simulink model "double_inverted_pendulum3"  (R2021b)
settings: Solver=VariableStepAuto  StartTime=0.0  StopTime=20  RelTol=1e-3
libraries: mpclib x1
settings Model: Creator=Dev Vaibhav  LastModifiedBy=Dev Vaibhav

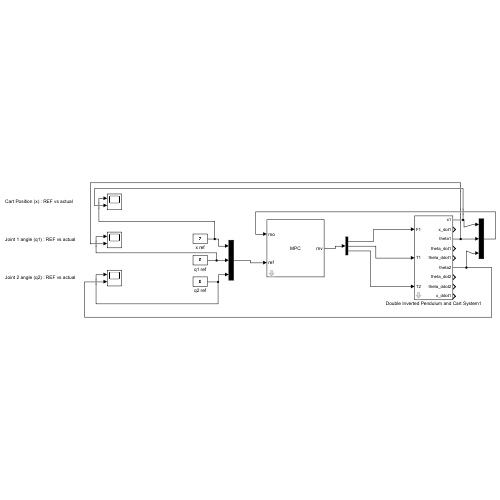
[thumbnail: Simulink's stored preview of the top-level diagram]
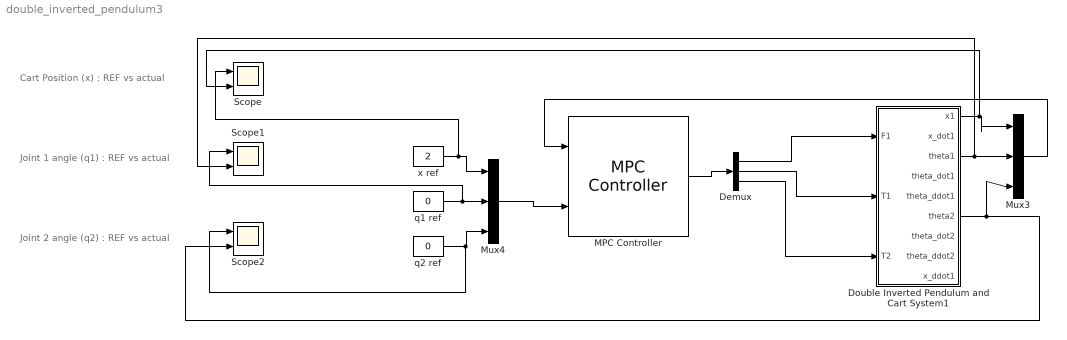
== system double_inverted_pendulum3 ==
  note: Cart Position (x) : REF vs actual
  note: Joint 1 angle (q1) : REF vs actual
  note: Joint 2 angle (q2) : REF vs actual
  Demux : Demux  Outputs=3
  Double Inverted Pendulum and Cart System1 : Subsystem  mask{mCartPara=1, mPendPara=1, gPara=9.81, LPara=0.5, KdPara=10}
      mask prompts: mCartPara "Mass of Cart"; mPendPara "Mass of Pendulum"; gPara "Gravity"; LPara "Length of Pendulum"; KdPara "Friction coefficient of Cart"
      mask help: Pendulum and Cart System
      mask init:
      | mCart = str2double(get_param(gcb,'mCartPara'));
      | mPend = str2double(get_param(gcb,'mPendPara'));
      | g = str2double(get_param(gcb,'gPara'));
      | L = str2double(get_param(gcb,'LPara'));
      | Kd = str2double(get_param(gcb,'KdPara'));
  MPC Controller : mpclib/MPC Controller  SCDEnableBlockLinearizationSpecification=on  mpcobj=mpc1  is_multiple=0  enable_value=0  return_u0=off  updateMPCinCallerWorkspace=on  md_inport=off  mv_inport=off  uref_inport=off  return_cost=off  return_mvseq=off  return_qpstatus=off  return_xseq=off  return_state=off  return_ovseq=off  state_inport=off  umin_inport=off  umax_inport=off  ymin_inport=off  ymax_inport=off  cc_inport=off  ywt_inport=off  uwt_inport=off  duwt_inport=off  rhoeps_inport=off  pm_inport=off  MaximumP=10  HorizonChoice=FixedHorizon  n_ts=0.05  n_p=13  n_mv=3  n_md=0  n_ud=0  n_mo=3  n_uo=0  BlockDataType=double  SampleTimeInherited=off  switch_inport=off
  Mux3 : Mux  Inputs=3
  Mux4 : Mux  Inputs=3
  Scope : Scope  NumInputPorts=2
  Scope1 : Scope  NumInputPorts=2
  Scope2 : Scope  NumInputPorts=2
  q1 ref : Constant  Value=0
  q2 ref : Constant  Value=0
  x ref : Constant  Value=2
  wires:
  q1 ref/1 -> Scope1/1, Mux4/2
  Demux/3 -> Double Inverted Pendulum and Cart System1/3(T2)
  MPC Controller/1 -> Demux/1
  Mux3/1 -> MPC Controller/1
  Demux/2 -> Double Inverted Pendulum and Cart System1/2(T1)
  Demux/1 -> Double Inverted Pendulum and Cart System1/1(F1)
  Double Inverted Pendulum and Cart System1/1(x1) -> Scope/2, Mux3/1
  Double Inverted Pendulum and Cart System1/3(theta1) -> Scope1/2, Mux3/2
  q2 ref/1 -> Scope2/1, Mux4/3
  Mux4/1 -> MPC Controller/2
  x ref/1 -> Scope/1, Mux4/1
  Double Inverted Pendulum and Cart System1/6(theta2) -> Scope2/2, Mux3/3

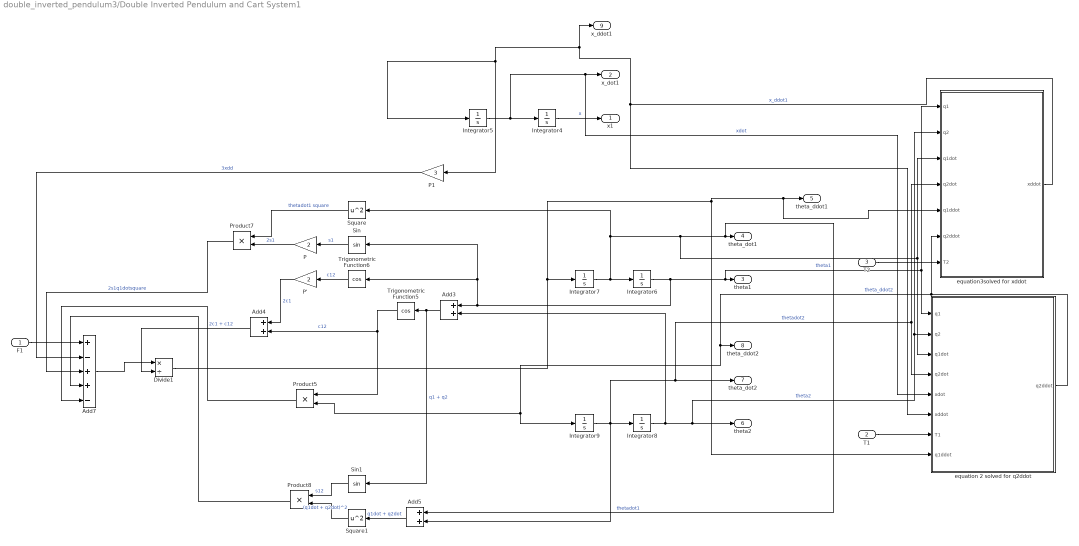
== system double_inverted_pendulum3/Double Inverted Pendulum and Cart System1 ==
  F1 : Inport
  T1 : Inport  Port=2
  T2 : Inport  Port=3
  Add3 : Sum
  Add4 : Sum
  Add5 : Sum
  Add7 : Sum  Inputs=+-++-
  Divide1 : Product  Inputs=*/
  Integrator4 : Integrator  ContinuousStateAttributes='x'
  Integrator5 : Integrator  ContinuousStateAttributes='xdot'
  Integrator6 : Integrator  ContinuousStateAttributes='theta'
  Integrator7 : Integrator  ContinuousStateAttributes='thetadot'
  Integrator8 : Integrator  ContinuousStateAttributes='theta'
  Integrator9 : Integrator  ContinuousStateAttributes='thetadot'
  P : Gain  Gain=2
  P' : Gain  Gain=2
  P1 : Gain  Gain=3
  Product5 : Product
  Product7 : Product
  Product8 : Product
  Sin : Trigonometry
  Sin1 : Trigonometry
  Square : Math  Operator=square  SaturateOnIntegerOverflow=on
  Square1 : Math  Operator=square  SaturateOnIntegerOverflow=on
  Trigonometric Function5 : Trigonometry  Operator=cos
  Trigonometric Function6 : Trigonometry  Operator=cos
  equation 2 solved for q2ddot : Subsystem
  equation3solved for xddot : Subsystem
  x1 : Outport  VectorParamsAs1DForOutWhenUnconnected=off
  x_dot1 : Outport  Port=2  VectorParamsAs1DForOutWhenUnconnected=off
  theta1 : Outport  Port=3  VectorParamsAs1DForOutWhenUnconnected=off
  theta_dot1 : Outport  Port=4  VectorParamsAs1DForOutWhenUnconnected=off
  theta_ddot1 : Outport  Port=5  VectorParamsAs1DForOutWhenUnconnected=off
  theta2 : Outport  Port=6  VectorParamsAs1DForOutWhenUnconnected=off
  theta_dot2 : Outport  Port=7  VectorParamsAs1DForOutWhenUnconnected=off
  theta_ddot2 : Outport  Port=8  VectorParamsAs1DForOutWhenUnconnected=off
  x_ddot1 : Outport  Port=9  VectorParamsAs1DForOutWhenUnconnected=off
  wires:
  Integrator7/1 -> Integrator6/1, Square/1, equation3solved for xddot/3(q1dot), equation 2 solved for q2ddot/3(q1dot), Add5/1, theta_dot1/1  "thetadot1"
  equation3solved for xddot/1(xddot) -> P1/1, Integrator5/1, x_ddot1/1, equation 2 solved for q2ddot/6(xddot)  "x_ddot1"
  Integrator5/1 -> equation 2 solved for q2ddot/5(xdot), x_dot1/1, Integrator4/1  "xdot"
  Integrator6/1 -> Sin/1, Trigonometric Function6/1, Add3/1, equation 2 solved for q2ddot/1(q1), equation3solved for xddot/1(q1), theta1/1  "theta1"
  Integrator4/1 -> x1/1  "x"
  Integrator9/1 -> Add5/2, Integrator8/1, equation3solved for xddot/4(q2dot), equation 2 solved for q2ddot/4(q2dot), theta_dot2/1  "thetadot2"
  Integrator8/1 -> Add3/2, equation3solved for xddot/2(q2), equation 2 solved for q2ddot/2(q2), theta2/1  "theta2"
  equation 2 solved for q2ddot/1(q2ddot) -> Integrator9/1, Product5/2, theta_ddot2/1, equation3solved for xddot/6(q2ddot)  "theta_ddot2"
  Add3/1 -> Sin1/1, Trigonometric Function5/1  "q1 + q2"
  Trigonometric Function5/1 -> Add4/2, Product5/1  "c12"
  Trigonometric Function6/1 -> P'/1  "c12"
  P'/1 -> Add4/1  "2c1"
  Sin/1 -> P/1  "s1"
  P/1 -> Product7/2  "2s1"
  Square/1 -> Product7/1  "thetadot1 square"
  Add5/1 -> Square1/1  "q1dot + q2dot"
  Square1/1 -> Product8/2  "(q1dot + q2dot)^2"
  Sin1/1 -> Product8/1  "s12"
  Product8/1 -> Add7/4
  Product7/1 -> Add7/3  "2s1q1dotsquare"
  F1/1 -> Add7/1
  P1/1 -> Add7/2  "3xdd"
  Product5/1 -> Add7/5
  Add7/1 -> Divide1/1
  Add4/1 -> Divide1/2  "2c1 + c12"
  T1/1 -> equation 2 solved for q2ddot/7(T1)
  T2/1 -> equation3solved for xddot/7(T2)
  Divide1/1 -> equation 2 solved for q2ddot/8(q1ddot), equation3solved for xddot/5(q1ddot), theta_ddot1/1, Integrator7/1

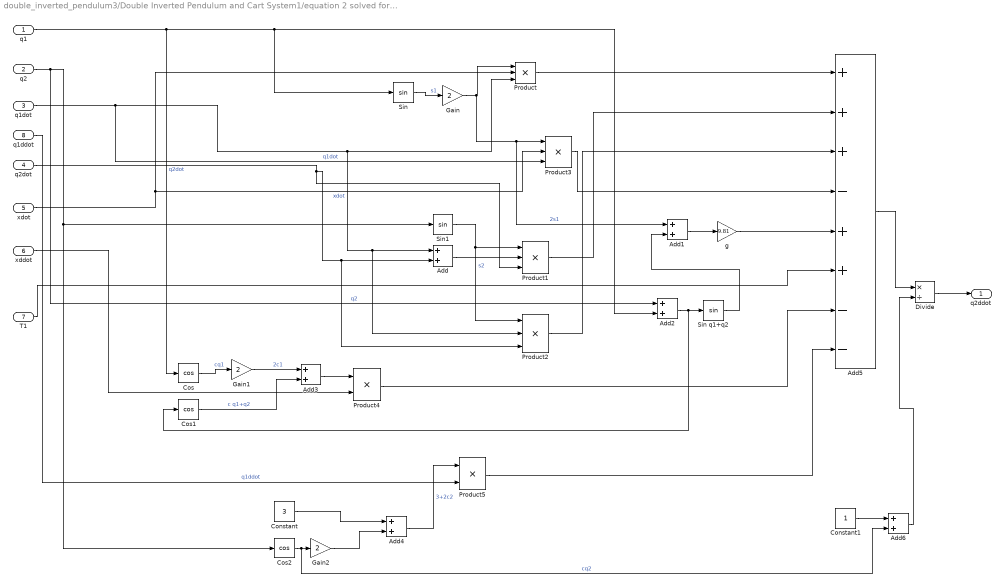
== system double_inverted_pendulum3/Double Inverted Pendulum and Cart System1/equation 2 solved for q2ddot ==
  q1 : Inport
  q2 : Inport  Port=2
  q1dot : Inport  Port=3
  q2dot : Inport  Port=4
  xdot : Inport  Port=5
  xddot : Inport  Port=6
  T1 : Inport  Port=7
  q1ddot : Inport  Port=8
  Add{,1..4,6} (6 alike) : Sum
  Add5 : Sum  Inputs=+++-++--
  Constant : Constant  Value=3
  Constant1 : Constant
  Cos : Trigonometry  Operator=cos
  Cos1 : Trigonometry  Operator=cos
  Cos2 : Trigonometry  Operator=cos
  Divide : Product  Inputs=*/
  Gain : Gain  Gain=2
  Gain1 : Gain  Gain=2
  Gain2 : Gain  Gain=2
  Product{,1..3} (4 alike) : Product  Inputs=3
  Product4 : Product
  Product5 : Product
  Sin : Trigonometry
  Sin q1+q2 : Trigonometry
  Sin1 : Trigonometry
  g : Gain  Gain=9.81
  q2ddot : Outport
  wires:
  q1/1 -> Cos/1, Add2/2, Sin/1
  Sin/1 -> Gain/1  "s1"
  Gain/1 -> Add1/1, Product3/1, Product/1  "2s1"
  xdot/1 -> Product3/2, Product/2  "xdot"
  q2/1 -> Add2/1, Cos2/1, Sin1/1  "q2"
  q2dot/1 -> Product1/3, Product2/3, Add/2  "q2dot"
  Sin1/1 -> Product2/1, Product1/1  "s2"
  Add/1 -> Product1/2
  q1dot/1 -> Product3/3, Product2/2, Add/1, Product/3  "q1dot"
  Add2/1 -> Cos1/1, Sin q1+q2/1
  Sin q1+q2/1 -> Add1/2
  Add1/1 -> g/1
  Cos/1 -> Gain1/1  "cq1"
  Gain1/1 -> Add3/1  "2c1"
  Cos1/1 -> Add3/2  "c q1+q2"
  Add3/1 -> Product4/1
  xddot/1 -> Product4/2
  Cos2/1 -> Add6/2, Gain2/1  "cq2"
  Constant/1 -> Add4/1
  Gain2/1 -> Add4/2
  Add4/1 -> Product5/1  "3+2c2"
  q1ddot/1 -> Product5/2  "q1ddot"
  Product/1 -> Add5/1
  Product1/1 -> Add5/2
  Product2/1 -> Add5/3
  Product3/1 -> Add5/4
  g/1 -> Add5/5
  T1/1 -> Add5/6
  Product4/1 -> Add5/7
  Product5/1 -> Add5/8
  Add5/1 -> Divide/1
  Constant1/1 -> Add6/1
  Add6/1 -> Divide/2
  Divide/1 -> q2ddot/1

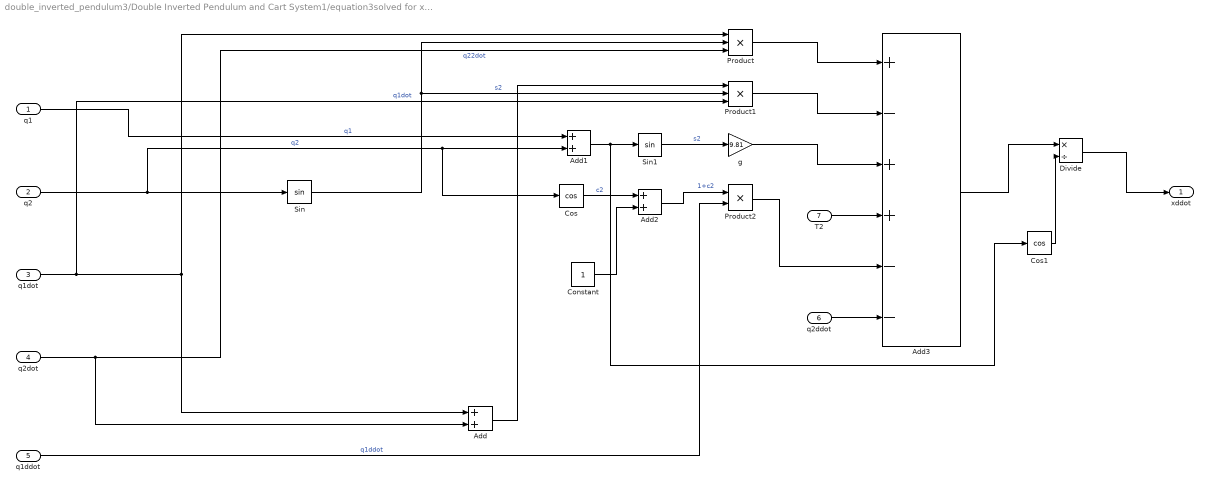
== system double_inverted_pendulum3/Double Inverted Pendulum and Cart System1/equation3solved for xddot ==
  q1 : Inport
  q2 : Inport  Port=2
  q1dot : Inport  Port=3
  q2dot : Inport  Port=4
  q1ddot : Inport  Port=5
  q2ddot : Inport  Port=6
  T2 : Inport  Port=7
  Add : Sum
  Add1 : Sum
  Add2 : Sum
  Add3 : Sum  Inputs=+-++--
  Constant : Constant
  Cos : Trigonometry  Operator=cos
  Cos1 : Trigonometry  Operator=cos
  Divide : Product  Inputs=*/
  Product : Product  Inputs=3
  Product1 : Product  Inputs=3
  Product2 : Product
  Sin : Trigonometry
  Sin1 : Trigonometry
  g : Gain  Gain=9.81
  xddot : Outport
  wires:
  q2/1 -> Cos/1, Add1/2, Sin/1  "q2"
  Sin/1 -> Product1/2, Product/2  "s2"
  q1dot/1 -> Product1/3, Add/1, Product/1  "q1dot"
  q2dot/1 -> Add/2, Product/3  "q22dot"
  Add/1 -> Product1/1
  q1/1 -> Add1/1  "q1"
  Add1/1 -> Cos1/1, Sin1/1
  Sin1/1 -> g/1  "s2"
  Cos/1 -> Add2/1  "c2"
  Constant/1 -> Add2/2
  Add2/1 -> Product2/1  "1+c2"
  q1ddot/1 -> Product2/2  "q1ddot"
  Product/1 -> Add3/1
  Product1/1 -> Add3/2
  g/1 -> Add3/3
  T2/1 -> Add3/4
  Product2/1 -> Add3/5
  q2ddot/1 -> Add3/6
  Cos1/1 -> Divide/2
  Add3/1 -> Divide/1
  Divide/1 -> xddot/1
